simulink model "model_pin"  (R2020a)
settings: Solver=VariableStepAuto  StartTime=0.0  StopTime=1000  RelTol=1e-3  EnableMultiTasking=on
undefined symbols (not defined in the file or in its folder): params
settings Model: Creator=user  LastModifiedBy=user
settings DataIOCC: ReturnWorkspaceOutputs=off
settings OptimizationCC: LifeSpan=inf
settings DebuggingCC: SFUnexpectedBacktrackingDiag=warning  SFNoUnconditionalDefaultTransitionDiag=warning  ArithmeticOperatorsInVariantConditions=warning
settings SFSimCC: SimUseLocalCustomCode=off  CustomCodeUndefinedFunction=UseInterfaceOnly
settings RTWCC: RTWUseLocalCustomCode=off
settings CodeAppCC: StateflowObjectComments=on
settings GRTTargetCC: TargetLangStandard=C89/C90 (ANSI)
settings ConfigComp: CovMetricSettings=dw  CovHtmlReporting=on  CovSaveCumulativeToWorkspaceVar=on  CovSaveSingleToWorkspaceVar=on  CovExternalEMLEnable=off

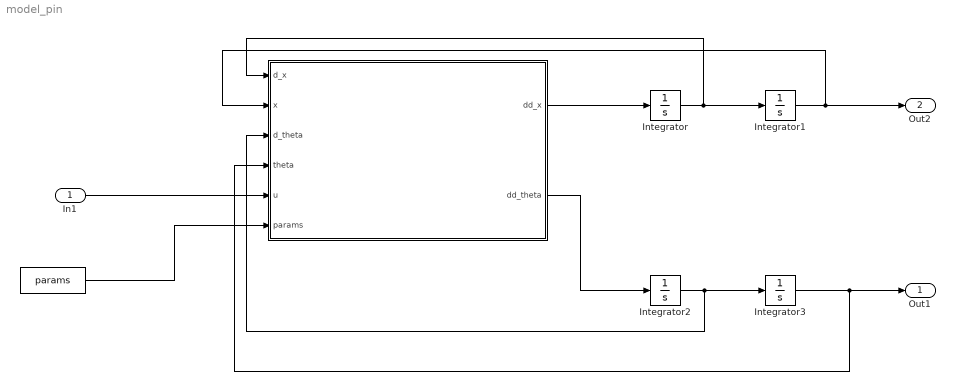
== system model_pin ==
  In1 : Inport
  " " : Constant  Value=params  OutDataTypeStr=Bus: params_bus
  " " : MATLAB Function  TreatAsAtomicUnit=on
  Integrator{,1..3} (4 alike) : Integrator
  Out1 : Outport
  Out2 : Outport  Port=2
  wires:
  " "/1(dd_x) -> Integrator/1
  " "/2(dd_theta) -> Integrator2/1
  Integrator/1 -> Integrator1/1, " "/1(d_x)
  Integrator2/1 -> Integrator3/1, " "/3(d_theta)
  In1/1 -> " "/5(u)
  " "/1 -> " "/6(params)
  Integrator3/1 -> Out1/1, " "/4(theta)
  Integrator1/1 -> Out2/1, " "/2(x)

== matlab function model_pin/  ==
  data: d_x input; x input; d_theta input; theta input; u input; dd_x output; params input; dd_theta output
function [dd_x, dd_theta] = fcn(d_x, x, d_theta, theta, u, params)
    dd_x = params.l * (d_theta)^2 - (params.k*x)/params.m + params.g*cos(theta) - params.zeta * d_x;
    dd_theta = (-params.g*sin(theta))/params.l - (2 * d_x * d_theta)/params.l - params.zeta * d_theta + u/(params.m * params.l^2);
%%y = u;
